simulink model "exam3"  (R2023a)
settings: Solver=FixedStepAuto  StartTime=0.0  StopTime=sim_time  FixedStep=sim_step  RelTol=1e-9
values from neighbouring files (symbols this model uses):
  D = 4.84812023585    [Derivative-bez-pokuty.mat]    (also in Derivative-pokuta.mat = 5.31896807598; IAE-obmedzenie1.mat = 4.3867984958; IAE-obmedzenie2.mat = 5.47171438855; UM4Sc.m = population(50,3))
  I = 17.7224780048    [Derivative-bez-pokuty.mat]    (also in Derivative-pokuta.mat = 17.2229129899; IAE-obmedzenie1.mat = 16.5552072014; IAE-obmedzenie2.mat = 17.6708327191; UM4Sc.m = population(50,2))
  P = 21.92628715    [Derivative-bez-pokuty.mat]    (also in Derivative-pokuta.mat = 23.6380434019; IAE-obmedzenie1.mat = 18.9460154326; IAE-obmedzenie2.mat = 26.4127638782; UM4Sc.m = population(50,1))
libraries: slpidlib x1, SignalEditorBlockLib x1
settings Model: Creator=laptop  LastModifiedBy=laptop

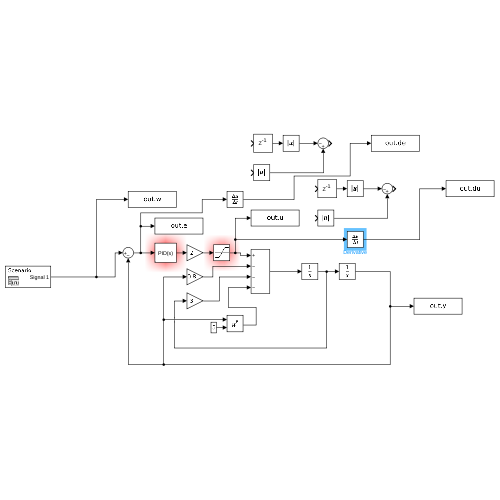
[thumbnail: Simulink's stored preview of the top-level diagram]
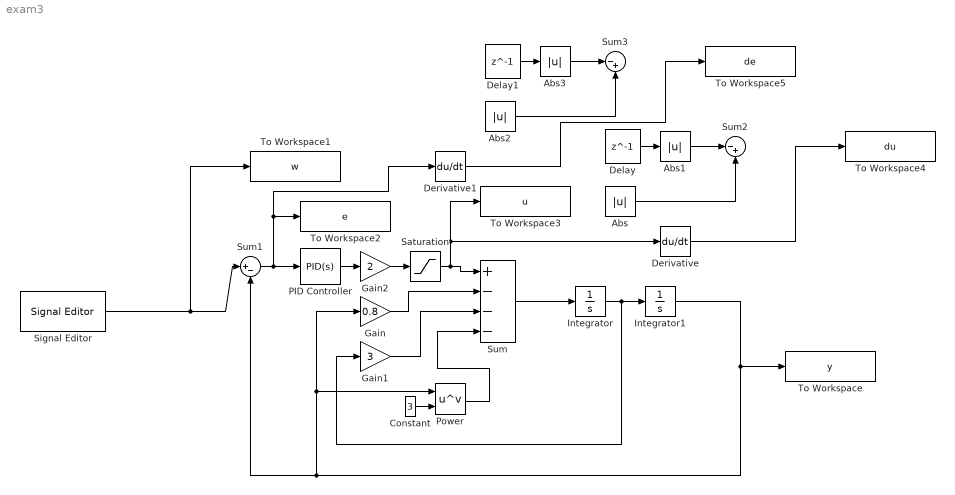
== system exam3 ==
  Abs{,1..3} (4 alike) : Abs  SaturateOnIntegerOverflow=off
  Constant : Constant  Value=3
  Delay : Delay  DelayLength=1
  Delay1 : Delay  DelayLength=1
  Derivative : Derivative
  Derivative1 : Derivative
  Gain : Gain  Gain=0.8
  Gain1 : Gain  Gain=3
  Gain2 : Gain  Gain=2
  Integrator : Integrator
  Integrator1 : Integrator
  PID Controller : slpidlib/PID Controller  Controller=PID  Form=Parallel  TimeDomain=Continuous-time  UseExternalTs=off  SampleTime=-1  IntegratorMethod=Forward Euler  FilterMethod=Forward Euler  ControllerParametersSource=internal  P=P  I=I  UseKiTs=off  D=D  N=100  UseFilter=on  TunerSelectOption=Transfer Function Based (PID Tuner App)  InitialConditionSource=internal  InitialConditionForIntegrator=0  InitialConditionForFilter=0  DifferentiatorICPrevScaledInput=0  ExternalReset=none  TrackingMode=off  Kt=1  LimitOutput=off  SatLimitsSource=internal  UpperSaturationLimit=inf  LowerSaturationLimit=-inf  LinearizeAsGain=on  AntiWindupMode=none  Kb=1  LimitIntegrator=off  UpperIntegratorSaturationLimit=inf  LowerIntegratorSaturationLimit=-inf  POutMin=[]  POutMax=[]  IOutMin=[]  IOutMax=[]  DOutMin=[]  DOutMax=[]  NOutMin=[]  NOutMax=[]  SumOutMin=[]  SumOutMax=[]  SaturationOutMin=[]  SaturationOutMax=[]  PParamMin=[]  PParamMax=[]  IParamMin=[]  IParamMax=[]  DParamMin=[]  DParamMax=[]  NParamMin=[]  NParamMax=[]  KbParamMin=[]  KbParamMax=[]  KtParamMin=[]  KtParamMax=[]  KbOutMin=[]  KbOutMax=[]  KtOutMin=[]  KtOutMax=[]  IntegratorOutMin=[]  IntegratorOutMax=[]  FilterOutMin=[]  FilterOutMax=[]  SumI1OutMin=[]  SumI1OutMax=[]  SumI2OutMin=[]  SumI2OutMax=[]  SumI3OutMin=[]  SumI3OutMax=[]  SumI4OutMin=[]  SumI4OutMax=[]  SumDOutMin=[]  SumDOutMax=[]  DifferentiatorOutMin=[]  DifferentiatorOutMax=[]  FilterDiffOutCoefMin=[]  FilterDiffOutCoefMax=[]  ReciprocalOutMin=[]  ReciprocalOutMax=[]  SumDenOutMin=[]  SumDenOutMax=[]  SumNumOutMin=[]  SumNumOutMax=[]  DivideOutMin=[]  DivideOutMax=[]  UdiffTsProdOutMin=[]  UdiffTsProdOutMax=[]  NTsProdOutMin=[]  NTsProdOutMax=[]  UintegralTsProdOutMin=[]  UintegralTsProdOutMax=[]  UngainTsProdOutMin=[]  UngainTsProdOutMax=[]  ClampingZeroOutDataTypeStr=Inherit: Inherit via back propagation  ClampingZeroOutMin=[]  ClampingZeroOutMax=[]  FilterDenConstantOutDataTypeStr=Inherit: Inherit via back propagation  FilterDenConstantOutMin=[]  FilterDenConstantOutMax=[]  PCopyOutDataTypeStr=Inherit: Inherit via back propagation  PCopyOutMin=[]  PCopyOutMax=[]  NCopyOutDataTypeStr=Inherit: Inherit via back propagation  NCopyOutMin=[]  NCopyOutMax=[]  IntegratorContinuousStateAttributes=''  IntegratorStateMustResolveToSignalObject=off  IntegratorRTWStateStorageClass=Auto  FilterContinuousStateAttributes=''  FilterStateMustResolveToSignalObject=off  FilterRTWStateStorageClass=Auto  ParallelPVariant=InternalParameters  IdealPVariant=Disabled  IVariant=InternalParameters  DVariant=InternalParameters  IntegratorVariant=Continuous  SatVariant=Disabled  AWVariant=Passthrough  PCopyVariant=Disabled  TRVariant=Disabled  FdbkBlocksVariant=Forward  IdealPFdbkVariant=Disabled  SatFdbkVariant=Disabled  DerivativeFilterVariant=ContFilter  NVariant=InternalParameters  NCopyVariant=Disabled  FilterICVariant=InternalICsFilter  IntegratorICVariant=InternalICs  ExternalResetVariant=Disabled  TRSumVariant=Passthrough  SumFdbkVariant=Disabled  SumVariant=Sum_PID  TsampFilterVariant=InternalTs  TsampNgainVariant=Passthrough  TsampIntegralVariant=Disabled_SignalSpec  ExternalSaturationOutDataTypeStr=Inherit: Same as second input
  Power : Math  Operator=pow
  Saturation : Saturate  UpperLimit=2*u  LowerLimit=-2*u
  Signal Editor : SignalEditorBlockLib/Signal Editor  FileName=signalmat.mat  ActiveScenario=Scenario  ActiveSignal=Signal 1  IsBus=off  OutputBusObjectStr=Bus: BusObject  SampleTime=0  Interpolate=off  ZeroCross=off  OutputAfterFinalValue=Holding final value  Unit=inherit  PreserveSignalName=on  ApplySigPropsToAllScenarios=on
  Sum : Sum  Inputs=+---
  Sum1 : Sum  Inputs=|+-
  Sum2 : Sum  Inputs=|-+
  Sum3 : Sum  Inputs=|-+
  To Workspace : ToWorkspace  VariableName=y  SaveFormat=Timeseries  SampleTime=-1
  To Workspace1 : ToWorkspace  VariableName=w  SaveFormat=Timeseries  SampleTime=-1
  To Workspace2 : ToWorkspace  VariableName=e  SaveFormat=Timeseries  SampleTime=-1
  To Workspace3 : ToWorkspace  VariableName=u  SaveFormat=Timeseries  SampleTime=-1
  To Workspace4 : ToWorkspace  VariableName=du  SaveFormat=Timeseries  SampleTime=-1
  To Workspace5 : ToWorkspace  VariableName=de  SaveFormat=Timeseries  SampleTime=-1
  wires:
  Gain/1 -> Sum/2
  Gain1/1 -> Sum/3
  Integrator/1 -> Gain1/1, Integrator1/1
  Power/1 -> Sum/4
  Integrator1/1 -> Gain/1, Power/1, Sum1/2, To Workspace/1
  Constant/1 -> Power/2
  Sum/1 -> Integrator/1
  Saturation/1 -> Derivative/1, To Workspace3/1, Sum/1
  Sum1/1 -> Derivative1/1, To Workspace2/1, PID Controller/1
  Signal Editor/1 -> To Workspace1/1, Sum1/1
  PID Controller/1 -> Gain2/1
  Gain2/1 -> Saturation/1
  Delay/1 -> Abs1/1
  Abs1/1 -> Sum2/1
  Abs/1 -> Sum2/2
  Delay1/1 -> Abs3/1
  Abs3/1 -> Sum3/1
  Abs2/1 -> Sum3/2
  Derivative1/1 -> To Workspace5/1
  Derivative/1 -> To Workspace4/1
